simulink model "DSSS_jamming"  (Simulink 8.7)
settings: Solver=ode45  StartTime=0.0  StopTime=inf  RelTol=1e-3
libraries: commdigbbndam3 x4, commchan3 x2, commsink2 x2, commrandsrc2 x2, dspindex x2, dspsrcs4 x2, commseqgen2 x1, commfilt2 x1, commutil2 x1
settings Model: Creator=Jinwoo Kim  LastModifiedBy=Administrator
settings DataIOCC: SignalLoggingSaveFormat=ModelDataLogs
settings OptimizationCC: ExpressionDepthLimit=2147483647  InitFltsAndDblsToZero=on
settings DebuggingCC: SaveWithParameterizedLinksMsg=none  SignalResolutionControl=TryResolveAllWithWarning  SolverPrmCheckMsg=warning  MultiTaskDSMMsg=warning  MultiTaskCondExecSysMsg=none  FcnCallInpInsideContextMsg=UseLocalSettings  StateNameClashWarn=warning
settings GRTTargetCC: TargetFcnLib=ansi_tfl_tmw.mat  CombineOutputUpdateFcns=off  GRTInterface=on

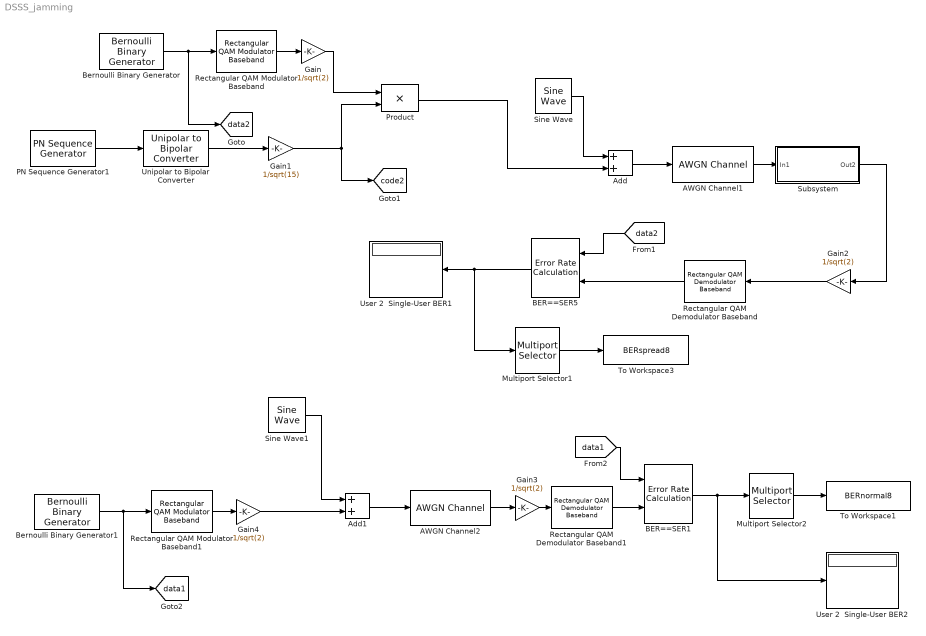
== system DSSS_jamming ==
  AWGN Channel1 : commchan3/AWGN Channel  InputProcessing=Inherited (this choice will be removed - see release notes)  seed=67  noiseMode="Signal to noise ratio  (Eb/No)"  EbNodB=10  EsNodB=10  SNRdB=7  bitsPerSym=30  Ps=1  Tsym=1e-3  variance=1
  AWGN Channel2 : commchan3/AWGN Channel  InputProcessing=Inherited (this choice will be removed - see release notes)  seed=67  noiseMode="Signal to noise ratio  (Eb/No)"  EbNodB=10  EsNodB=10  SNRdB=7  bitsPerSym=2  Ps=1  Tsym=1e-3  variance=1
  Add : Sum
  Add1 : Sum
  BER==SER1 : commsink2/Error Rate Calculation  N=0  st_delay=0  cp_mode=Entire frame  subframe=[]  PMode=Port  WsName=ErrorVec  RsMode2=off  stop=off  numErr=100  maxBits=1e6
  BER==SER5 : commsink2/Error Rate Calculation  N=0  st_delay=0  cp_mode=Entire frame  subframe=[]  PMode=Port  WsName=ErrorVec  RsMode2=off  stop=off  numErr=100  maxBits=1e6
  Bernoulli Binary Generator : commrandsrc2/Bernoulli Binary Generator  P=0.5  seed=61  Ts=1e-3/2  frameBased=on  sampPerFrame=2  orient=off  outDataType=double
  Bernoulli Binary Generator1 : commrandsrc2/Bernoulli Binary Generator  P=0.5  seed=61  Ts=1e-3/2  frameBased=on  sampPerFrame=2  orient=off  outDataType=double
  Gain{,2..4} (4 alike) : Gain  Gain=1/sqrt(2)  SaturateOnIntegerOverflow=on
  Gain1 : Gain  Gain=1/sqrt(15)  SaturateOnIntegerOverflow=on
  Multiport Selector1 : dspindex/Multiport Selector  rowsOrCols=Rows  idxCellArray={1}  idxErrMode=Clip Index
  Multiport Selector2 : dspindex/Multiport Selector  rowsOrCols=Rows  idxCellArray={1}  idxErrMode=Clip Index
  PN Sequence Generator1 : commseqgen2/PN Sequence Generator  poly=[1 1 0 0 1]  ini_sta=[0 0 0 1]  outBitMaskSource=Dialog parameter  shift=0  outVarSiz=off  maxOutSizeMode=Dialog parameter  maxOutSize=[10 1]  Ts=1e-3/15  frameBased=on  sampPerFrame=15  reset=off  bitPackedOutputs=off  outDataType=double  numPackedBits=8  bitPackDataSigned=off  bitPackedOutDType=double
  Product : Product  SaturateOnIntegerOverflow=on  InputSameDT=on  OutDataTypeStr=Inherit: Same as first input
  Rectangular QAM Demodulator Baseband : commdigbbndam3/Rectangular QAM Demodulator Baseband  M=4  OutType=Bit  DecType=Hard decision  VarSource=Dialog  Variance=1  Dec=Gray  Mapping=[0:15]  PowType=Min. distance between symbols  MinDist=2  AvgPow=1  PeakPow=1  Ph=0  outDtype1=double  outDtype2=double  derotateFactorWordLen=16  derotateFactorDataTypeStr=Inherit: Same word length as input  derotateFactorLastDataTypeStr=Inherit: Same word length as input  denormFactorWordLen=16  denormFactorDataTypeStr=Inherit: Same word length as input  denormFactorLastDataTypeStr=Inherit: Same word length as input  prodOutWordLen=32  prodOutOverflowMode=Wrap  prodOutRoundingMode=Floor  prodOutOvFlMode=off  prodOutOvFlModeLastStrValue=off  sumWordLen=32
  Rectangular QAM Demodulator Baseband1 : commdigbbndam3/Rectangular QAM Demodulator Baseband  M=4  OutType=Bit  DecType=Hard decision  VarSource=Dialog  Variance=1  Dec=Gray  Mapping=[0:15]  PowType=Min. distance between symbols  MinDist=2  AvgPow=1  PeakPow=1  Ph=0  outDtype1=double  outDtype2=double  derotateFactorWordLen=16  derotateFactorDataTypeStr=Inherit: Same word length as input  derotateFactorLastDataTypeStr=Inherit: Same word length as input  denormFactorWordLen=16  denormFactorDataTypeStr=Inherit: Same word length as input  denormFactorLastDataTypeStr=Inherit: Same word length as input  prodOutWordLen=32  prodOutOverflowMode=Wrap  prodOutRoundingMode=Floor  prodOutOvFlMode=off  prodOutOvFlModeLastStrValue=off  sumWordLen=32
  Rectangular QAM Modulator Baseband : commdigbbndam3/Rectangular QAM Modulator Baseband  M=4  InType=Bit  Enc=Gray  Mapping=[0:15]  PowType=Min. distance between symbols  MinDist=2  AvgPow=1  PeakPow=1  Ph=0  outDtype=double  outWordLen=16  outUDDataType=sfix(16)  outFracLenMode=Best precision  outFracLen=15  outDataTypeStr=double  outLastDataTypeStr=double
  Rectangular QAM Modulator Baseband1 : commdigbbndam3/Rectangular QAM Modulator Baseband  M=4  InType=Bit  Enc=Gray  Mapping=[0:15]  PowType=Min. distance between symbols  MinDist=2  AvgPow=1  PeakPow=1  Ph=0  outDtype=double  outWordLen=16  outUDDataType=sfix(16)  outFracLenMode=Best precision  outFracLen=15  outDataTypeStr=double  outLastDataTypeStr=double
  Sine Wave : dspsrcs4/Sine Wave  Amplitude=0.5  Frequency=250  Phase=0  SampleMode=Discrete  OutComplex=Complex  CompMethod=Trigonometric fcn  TableSize=Speed  SampleTime=1e-3  SamplesPerFrame=1  ResetState=Restart at time zero  OutputFrames=on  dataType=double  wordLen=16  udDataType=sfix(16)  fracBitsMode=Best precision  numFracBits=15  OutDataTypeStr=double  LastOutDataTypeStr=double
  Sine Wave1 : dspsrcs4/Sine Wave  Amplitude=0.5  Frequency=250  Phase=0  SampleMode=Discrete  OutComplex=Complex  CompMethod=Trigonometric fcn  TableSize=Speed  SampleTime=1e-3  SamplesPerFrame=1  ResetState=Restart at time zero  OutputFrames=on  dataType=double  wordLen=16  udDataType=sfix(16)  fracBitsMode=Best precision  numFracBits=15  OutDataTypeStr=double  LastOutDataTypeStr=double
  Subsystem : Subsystem
      mask Display: disp('Rx')
  To Workspace1 : ToWorkspace  VariableName=BERnormal8  SampleTime=-1
      settings: MaxDataPoints=1
  To Workspace3 : ToWorkspace  VariableName=BERspread8  SampleTime=-1
      settings: MaxDataPoints=1
  Unipolar to Bipolar Converter : commutil2/Unipolar to Bipolar Converter  M=2  polarity=Positive  dataType=Same as input
  User 2  Single-User BER1 : Display
  User 2  Single-User BER2 : Display
  tag scope: code2=global, data1=global, data2=global
  wires:
  AWGN Channel1/1 -> Subsystem/1(In1)
  Gain2/1 -> Rectangular QAM Demodulator Baseband/1
  [data2] -> BER==SER5/1
  Rectangular QAM Demodulator Baseband/1 -> BER==SER5/2
  BER==SER5/1 -> User 2  Single-User BER1/1, Multiport Selector1/1
  Subsystem/1(Out2) -> Gain2/1
  Multiport Selector1/1 -> To Workspace3/1
  Multiport Selector2/1 -> To Workspace1/1
  AWGN Channel2/1 -> Gain3/1
  Gain3/1 -> Rectangular QAM Demodulator Baseband1/1
  [data1] -> BER==SER1/1
  Rectangular QAM Demodulator Baseband1/1 -> BER==SER1/2
  BER==SER1/1 -> Multiport Selector2/1, User 2  Single-User BER2/1
  Gain/1 -> Product/1
  Gain1/1 -> Product/2, [code2]
  Rectangular QAM Modulator Baseband/1 -> Gain/1
  Bernoulli Binary Generator/1 -> Rectangular QAM Modulator Baseband/1, [data2]
  PN Sequence Generator1/1 -> Unipolar to Bipolar Converter/1
  Bernoulli Binary Generator1/1 -> [data1], Rectangular QAM Modulator Baseband1/1
  Rectangular QAM Modulator Baseband1/1 -> Gain4/1
  Add/1 -> AWGN Channel1/1
  Product/1 -> Add/2
  Add1/1 -> AWGN Channel2/1
  Gain4/1 -> Add1/2
  Sine Wave/1 -> Add/1
  Sine Wave1/1 -> Add1/1
  Unipolar to Bipolar Converter/1 -> Gain1/1

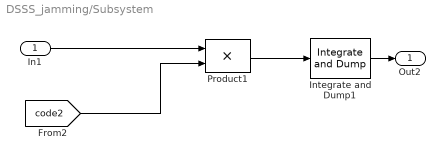
== system DSSS_jamming/Subsystem ==
  In1 : Inport
  Integrate and Dump1 : commfilt2/Integrate and Dump  obssamples=15  offsetsamples=0  nodump=off  roundingMode=Floor  overflowMode=off  outputDataTypeStr=Inherit: Same as accumulator  outputLastDataTypeStr=Inherit: Same as accumulator
  Product1 : Product  SaturateOnIntegerOverflow=on  InputSameDT=on  OutDataTypeStr=Inherit: Same as first input
  Out2 : Outport
  wires:
  Product1/1 -> Integrate and Dump1/1
  [code2] -> Product1/2
  In1/1 -> Product1/1
  Integrate and Dump1/1 -> Out2/1
